simulink model "MicroMouse_Deploy"  (R2024b)
settings: Solver=FixedStepAuto  StartTime=0.0  StopTime=inf  FixedStep=0.01  RelTol=1e-3  EnableMultiTasking=on
PreLoadFcn:
  | addpath(genpath(pwd))
  | 
  | MX_IOC_LOCATION = auto_MX_path()
undefined symbols (not defined in the file or in its folder): samplingTime
settings Model: STM32="{\"DigitalPortWrite\":[{\"ID\":\"newMicroMouseTemplate:84:3\"},{\"ID\":\"newMicroMouseTemplate:84:4\"},{\"ID\":\"newMicroMouseTemplate:84:5\"},{\"ID\":\"newMicroMouseTemplate:84:6\"},{\"ID\":\"newMicroMouseTemplate:84:7\"},{\"ID\":\"newMicroMouseTemplate:84:8\"},{\"ID\":\"newMicroMouseTemplate:84:9\"},{\"ID\":\"newMicroMouseTemplate:84:10\"}]}"  SimulationMode=external  ExtModeTrigDuration=10  Creator=JesseJabezArendse  LastModifiedBy=JesseJabezArendse
settings SolverCC: AllowMultiTaskInputOutput=on  AutoInsertRateTranBlk=on  InsertRTBMode=Never (minimum delay)
settings OptimizationCC: DefaultUnderspecifiedDataType=single  EnhancedBackFolding=on  PassReuseOutputArgsAs=Individual arguments  StateBitsets=on  DataBitsets=on  ZeroExternalMemoryAtStartup=off  ZeroInternalMemoryAtStartup=off  NoFixptDivByZeroProtection=on  MaxStackSize=4096  OptimizeBlockOrder=speed  DifferentSizesBufferReuse=on  EfficientTunableParamExpr=on
settings DebuggingCC: MultiTaskCondExecSysMsg=none  ParameterOverflowMsg=none  ParameterPrecisionLossMsg=none  ParameterTunabilityLossMsg=error
settings HardwareCC: ProdBitPerPointer=32  ProdBitPerSizeT=32  ProdBitPerPtrDiffT=32  ProdLargestAtomicInteger=Long  ProdLargestAtomicFloat=Double  ProdWordSize=32  ProdLongLongMode=on  ProdHWDeviceType=ARM Compatible->ARM Cortex  TargetBitPerPointer=64  TargetBitPerSizeT=64  TargetBitPerPtrDiffT=64  TargetLongLongMode=on  TargetIntDivRoundTo=Zero  TargetEndianess=LittleEndian  TargetWordSize=64  TargetHWDeviceType=MATLAB Host
settings ModelReferenceCC: UpdateModelReferenceTargets=AssumeUpToDate  EnableParallelModelReferenceBuilds=on  ParallelModelReferenceMATLABWorkerInit=Copy Base Workspace  SupportModelReferenceSimTargetCustomCode=on
settings SFSimCC: MATLABDynamicMemAlloc=off  SimHardwareAcceleration=native
settings RTWCC: Description=Embedded Coder  SystemTargetFile=ert.tlc  HardwareBoard=STM32L4xx Based  TLCOptions=-p0 -aInlineSetEventsForThisBaseRateFcn=TLC_FALSE -aSuppressMultiTaskScheduler=TLC_FALSE -aRateBasedStepFcn=1  TemplateMakefile=ert_default_tmf  RetainRTWFile=on  Toolchain=GNU Tools for ARM Embedded Processors  IncludeHyperlinkInReport=on  CodeExecutionProfiling=on  CodeProfilingInstrumentation=coarse  GPUComputeCapability=3.5
settings RTWCC: CustomHeaderCode=|
  | #include "MicroMouseProgramming_Code\Core\Inc\IMU.h"
  | #include "MicroMouseProgramming_Code\Core\Inc\Motors.h"
  | #include "MicroMouseProgramming_Code\Core\Inc\SSD1306.h"
  | #include "MicroMouseProgramming_Code\Core\Inc\VL53L0X.h"
  | #include "MicroMouseProgramming_Code\Core\Inc\ADCs.h"
  | #include "MicroMouseProgramming_Code\Core\Inc\Buttons.h"
  | #include "MicroMouseProgramming_Code\Core\Inc\LEDs.h"
  | #include "MicroMouseProgramming_Code\Core\Inc\INA219.h"
  | #include "MicroMouseProgramming_Code\Core\Inc\preformatted_flash.h"
settings RTWCC: CustomInclude=|
  | MicroMouseProgramming_Code\Core\Inc\
  | MicroMouseProgramming_Code\Core\Src\
  | MicroMouseProgramming_Code\Drivers\STM32L4xx_HAL_Driver\Inc\
  | MicroMouseProgramming_Code\Drivers\STM32L4xx_HAL_Driver\Src\
  | MicroMouseProgramming_Code\Drivers\CMSIS\Device\ST\STM32L4xx\Include\
  | MicroMouseProgramming_Code\Drivers\CMSIS\Core\Include\
settings RTWCC: CustomSource=|
  | MicroMouseProgramming_Code\Core\Src\IMU.c
  | MicroMouseProgramming_Code\Core\Src\Motors.c
  | MicroMouseProgramming_Code\Core\Src\SSD1306.c
  | MicroMouseProgramming_Code\Core\Src\VL53L0X.c
  | MicroMouseProgramming_Code\Core\Src\ADCs.c
  | MicroMouseProgramming_Code\Core\Src\Buttons.c
  | MicroMouseProgramming_Code\Core\Src\LEDs.c
  | MicroMouseProgramming_Code\Core\Src\INA219.c
  | MicroMouseProgramming_Code\Core\Src\preformatted_flash.c
settings RTWCC: CustomDefine=|
  | #define COMPILED_BY_SIMULINK
  | #define IMU_ICM42605
  | #define IMU_DYNAMIC_FSR
  | #define TOF_DYNAMIC_FSR
  | #define SCREEN_FONT_DYNAMIC
settings CodeAppCC: ForceParamTrailComments=on  IgnoreCustomStorageClasses=off  OperatorAnnotations=on  SimulinkDataObjDesc=on  SFDataObjDesc=on  InsertBlockDesc=on
settings ERTTargetCC: TargetLangStandard=C99 (ISO)  CodeReplacementLibrary=ARM Cortex-M  SupportNonFinite=off  SupportComplex=off  SupportContinuousTime=on  ExtModeTransport=3  ExtModeStaticAlloc=on  ExtModeStaticAllocSize=2048  ExtModeMexFile=ext_xcp  ExtModeIntrfLevel=Level2 - Open  InlinedParameterPlacement=Hierarchical  DynamicArrayContainerType=coder::array

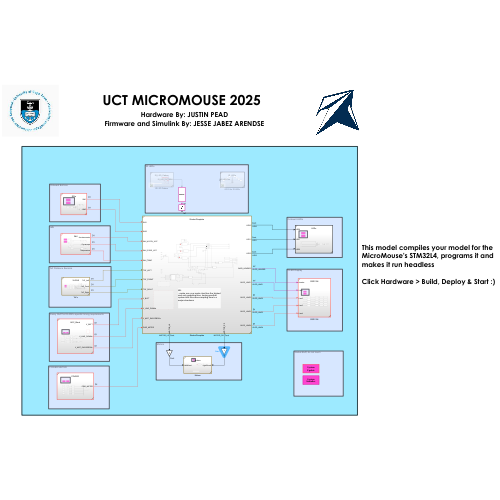
[thumbnail: Simulink's stored preview of the top-level diagram]
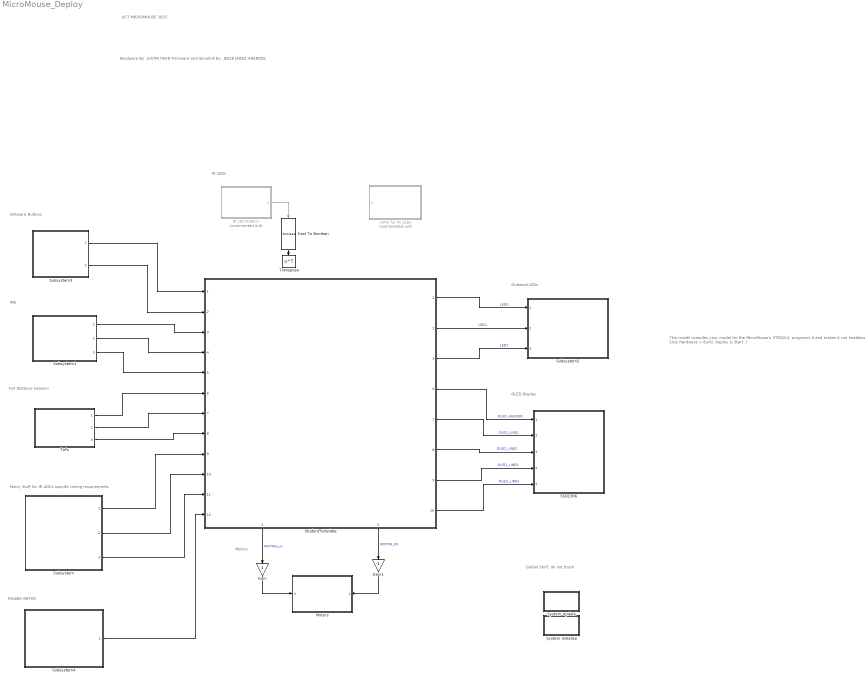
== system MicroMouse_Deploy ==
  note: POWER METER
  note: Global Stuff, do not touch
  note: OLED Display
  note: ToF Distance Sensors
  note: IMU
  note: Fancy Stuff for IR ADCs specific timing requirements
  note: IR LEDs
  note: Motors
  note: Onboard Buttons
  note: Onboard LEDs
  note: UCT MICROMOUSE 2025
  note: Hardware By: JUSTIN PEAD
      | Firmware and Simulink By: JESSE JABEZ ARENDSE
  note: This model compiles your model for the MicroMouse's STM32L4, programs it and makes it run headless
      |
      | Click Hardware > Build, Deploy & Start :)
  Cast To Boolean : DataTypeConversion  OutDataTypeStr=boolean  SaturateOnIntegerOverflow=off  RndMeth=Floor
  GPIO for IR LEDs : Subsystem  Commented=on  TreatAsAtomicUnit=on  SystemSampleTime=samplingTime  ReferencedSubsystem=IR_LEDs
  Gain : Gain  OutDataTypeStr=Inherit: Same as input
  Gain1 : Gain  Gain=-1  OutDataTypeStr=Inherit: Same as input
  IR LED Pattern : Subsystem  Commented=on  ReferencedSubsystem=IR_LED_Pattern
  Motors : Subsystem  ReferencedSubsystem=Motors
      settings: PortSchema="{\"entries\":[{\"content\":{\"sides\":[{\"content\":{\"connectorIds\":[\"In2\"]},\"type\":\"ConnectorPlacement.EquallySpacedRectSide\",\"uuid\":\"1d0b36bf-65cc-407d-99e2-9b57a669311c\"},{\"content\":{\"connectorIds\":[\"In1\"],\"side\":\"RIGHT\"},\"type\":\"ConnectorPlacement.EquallySpacedRectSide\",\"uuid\":\"0f431f71-a73a-435d-830e-9de719167e02\"},{\"content\":{\"side\":\"TOP\"},\"type\":\"ConnectorPlacement.EquallySpacedRectSide\",\"uuid\":\"bb39be10-7fb0-474e-8478-e15baad53e86\"}]},\"type\":\"ConnectorPlacement.EquallySpacedConnector\",\"uuid\":\"da48592d-6e4d-4f7f-85e6-7b017dfa5a37\"}],\"packageUris\":[\"http://schema.mathworks.com/mf0/Connector/R2020b\"],\"version\":\"1.0\"}"
  SSD1306 : Subsystem  ReferencedSubsystem=SSD1306
  StudentTemplate : Subsystem  ReferencedSubsystem=StudentTemplate
      settings: PortSchema="{\"entries\":[{\"content\":{\"sides\":[{\"content\":{\"connectorIds\":[\"In1\",\"In2\",\"In3\",\"In4\",\"In5\",\"In6\",\"In7\",\"In8\",\"In9\",\"In10\",\"In11\",\"In12\"]},\"type\":\"ConnectorPlacement.EquallySpacedRectSide\",\"uuid\":\"d1b9fe55-82ae-4911-bdae-d1742f45ad0b\"},{\"content\":{\"connectorIds\":[\"Out1\",\"Out2\",\"Out3\",\"Out6\",\"Out7\",\"Out8\",\"Out9\",\"Out10\"],\"side\":\"RIGHT\"},\"type\":\"ConnectorPlacement.EquallySpacedRectSide\",\"uuid\":\"a2268332-f9a7-4a23-904c-bb2af80d3f25\"},{\"content\":{\"side\":\"TOP\"},\"type\":\"ConnectorPlacement.EquallySpacedRectSide\",\"uuid\":\"b9258226-2626-4b1c-aaab-59e84007a065\"},{\"content\":{\"connectorIds\":[\"Out4\",\"Out5\"],\"side\":\"BOTTOM\"},\"type\":\"ConnectorPlacement.EquallySpacedRectSide\",\"uuid\":\"973b5380-9b77-47c6-ad42-ebf297573f24\"}]},\"type\":\"ConnectorPlacement.EquallySpacedConnector\",\"uuid\":\"d7520a25-4971-4993-9bed-0d1698e82bf0\"}],\"packageUris\":[\"http://schema.mathworks.com/mf0/Connector/R2020b\"],\"version\":\"1.0\"}"
  Subsystem : Subsystem  ReferencedSubsystem=ADC_Block
      settings: PortSchema="{\"entries\":[{\"content\":{\"sides\":[{\"content\":{},\"type\":\"ConnectorPlacement.EquallySpacedRectSide\",\"uuid\":\"97954fbc-a995-443d-a89d-5fc021da5850\"},{\"content\":{\"side\":\"RIGHT\"},\"type\":\"ConnectorPlacement.EquallySpacedRectSide\",\"uuid\":\"4d9d086b-245c-4f12-8434-deaa6fcb7387\"},{\"content\":{\"connectorIds\":[\"Out1\",\"Out2\",\"Out3\"],\"side\":\"TOP\"},\"type\":\"ConnectorPlacement.EquallySpacedRectSide\",\"uuid\":\"e3200828-6d34-4176-9821-d474c757d427\"}]},\"type\":\"ConnectorPlacement.EquallySpacedConnector\",\"uuid\":\"010323c9-37fe-4d77-99f8-4c689683127f\"}],\"packageUris\":[\"http://schema.mathworks.com/mf0/Connector/R2020b\"],\"version\":\"1.0\"}"
  Subsystem1 : Subsystem  ReferencedSubsystem=IMU
  Subsystem2 : Subsystem  ReferencedSubsystem=LEDs
  Subsystem3 : Subsystem  ReferencedSubsystem=SWs
  Subsystem4 : Subsystem  ReferencedSubsystem=POWER
  System Initialize : Subsystem  mask(System Initialize){ShowInLibBrowser=0}
      mask prompts: ShowInLibBrowser "Simulink:masks:CustCodeMaskParam1_MP"
      settings: CopyFcn=cccopyfcn(gcb)  OpenFcn=ccopenfcn('System Initialize Function')
      mask Help: eval('feval(''rtwprivate'',''rtwhelpview'',''rtw_sys_initialize_block'')');
      mask Display: disp('System\nInitialize');
  System Update : Subsystem  mask(System Update){ShowInLibBrowser=0}
      mask prompts: ShowInLibBrowser "Simulink:masks:CustCodeMaskParam1_MP"
      settings: CopyFcn=cccopyfcn(gcb)  OpenFcn=ccopenfcn('System Update Function')
      mask Help: eval('feval(''rtwprivate'',''rtwhelpview'',''rtw_sys_update_block'')');
      mask Display: disp('System\nUpdate');
  ToFs : Subsystem  ReferencedSubsystem=VL53L0
  Transpose : Math  Operator=transpose
  wires:
  Gain/1 -> Motors/2
  IR LED Pattern/1 -> Cast To Boolean/1
  Cast To Boolean/1 -> Transpose/1
  Subsystem3/1 -> StudentTemplate/1
  Subsystem3/2 -> StudentTemplate/2
  Subsystem1/1 -> StudentTemplate/3
  Subsystem1/2 -> StudentTemplate/4
  ToFs/1 -> StudentTemplate/6
  ToFs/2 -> StudentTemplate/7
  ToFs/3 -> StudentTemplate/8
  Subsystem/1 -> StudentTemplate/9
  Subsystem/2 -> StudentTemplate/10
  Subsystem/3 -> StudentTemplate/11
  StudentTemplate/1 -> Subsystem2/1  "LED0"
  StudentTemplate/2 -> Subsystem2/2  "LED1"
  StudentTemplate/3 -> Subsystem2/3  "LED2"
  StudentTemplate/4 -> Gain/1  "MOTOR_LS"
  StudentTemplate/5 -> Gain1/1  "MOTOR_RS"
  StudentTemplate/6 -> SSD1306/1  "OLED_HEADER"
  StudentTemplate/7 -> SSD1306/2  "OLED_LINE1"
  StudentTemplate/8 -> SSD1306/3  "OLED_LINE2"
  StudentTemplate/9 -> SSD1306/4  "OLED_LINE3"
  StudentTemplate/10 -> SSD1306/5  "OLED_LINE4"
  Subsystem1/3 -> StudentTemplate/5
  Subsystem4/1 -> StudentTemplate/12
  Gain1/1 -> Motors/1

== system MicroMouse_Deploy/System Initialize ==

== system MicroMouse_Deploy/System Update ==
